simulink model "realistic_model"  (R2021b)
settings: Solver=VariableStepAuto  StartTime=0.0  StopTime=10  RelTol=1e-3
values from neighbouring files (symbols this model uses):
  A = [0 0 1 0 ... (first row only)    [main.m]
  B = [0 ... (first row only)    [main.m]
  C = [1 0 0 0 ... (first row only)    [main.m]
  K = K_temp    [main.m]    (also in plots_assignment2.m; plots_assignment3.m)
  Ts = 0.05    [main.m]
  Wc = wc_temp    (= 12.5663706144)    [main.m]    (also in plots_assignment3.m = wc_temp; tuning.m = 40.8407044967)
  x_initial = [0 0 0 0]'    [main.m]    (also in tuning.m)
settings Model: Creator=Marius  LastModifiedBy=Marius

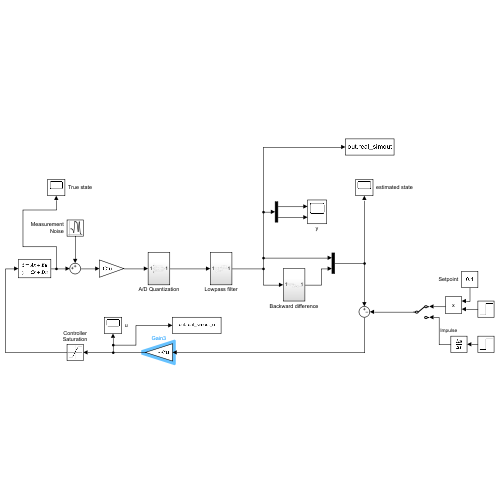
[thumbnail: Simulink's stored preview of the top-level diagram]
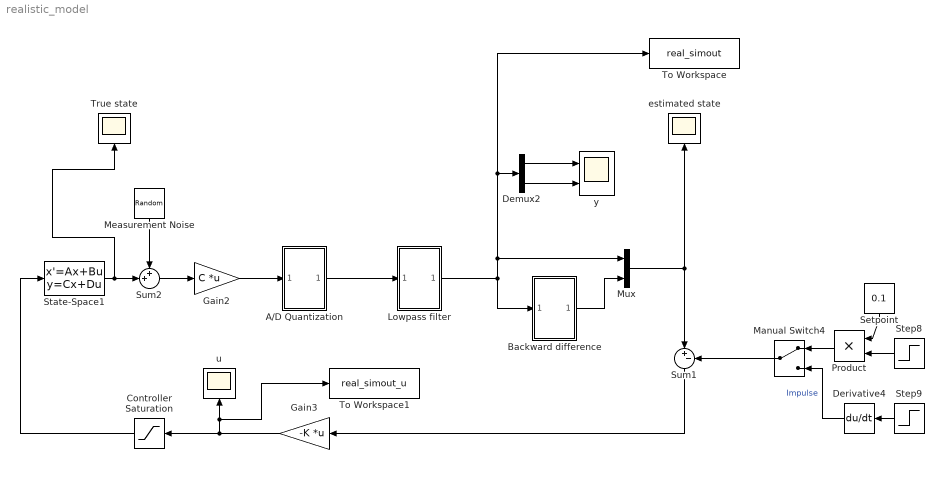
== system realistic_model ==
  A/D Quantization : Subsystem
  Backward difference : Subsystem
  Controller Saturation : Saturate  UpperLimit=5  LowerLimit=-5
  Demux2 : Demux  Outputs=2
  Derivative4 : Derivative
  Gain2 : Gain  Gain=C  Multiplication=Matrix(K*u)
  Gain3 : Gain  Gain=-K  Multiplication=Matrix(K*u)
  Lowpass filter : Subsystem
  Manual Switch4 : ManualSwitch
  Measurement Noise : RandomNumber  Mean=[0 0 0 0]  Variance=[0.0005 pi/1800 0 0].^2  SampleTime=0.1
  Mux : Mux  Inputs=2
  Product : Product
  Setpoint : Constant  Value=0.1
  State-Space1 : StateSpace  A=A  B=B  C=eye(4)  D=zeros(4,1)  InitialCondition=x_initial
  Step8 : Step  Before=[0 0 0 0]  After=[1 0 0 0]  SampleTime=0
  Step9 : Step  Before=[0 0 0 0]  After=[10 0 0 0]  SampleTime=0
  Sum1 : Sum  Inputs=|+-
  Sum2 : Sum  Inputs=++|
  To Workspace : ToWorkspace  VariableName=real_simout  SaveFormat=Timeseries  SampleTime=-1
  To Workspace1 : ToWorkspace  VariableName=real_simout_u  SaveFormat=Timeseries  SampleTime=-1
  True state : Scope
  estimated state : Scope
  u : Scope
  y : Scope  NumInputPorts=2
  wires:
  Manual Switch4/1 -> Sum1/2
  Gain3/1 -> Controller Saturation/1, To Workspace1/1, u/1
  Sum1/1 -> Gain3/1
  Demux2/2 -> y/2
  Demux2/1 -> y/1
  Step9/1 -> Derivative4/1
  Derivative4/1 -> Manual Switch4/2  "Impulse"
  Mux/1 -> estimated state/1, Sum1/1
  State-Space1/1 -> True state/1, Sum2/2
  Sum2/1 -> Gain2/1
  Measurement Noise/1 -> Sum2/1
  Backward difference/1(Out1) -> Mux/2
  Lowpass filter/1(Out1) -> Backward difference/1(In1), To Workspace/1, Demux2/1, Mux/1
  A/D Quantization/1(Out1) -> Lowpass filter/1(In1)
  Gain2/1 -> A/D Quantization/1(In1)
  Product/1 -> Manual Switch4/1
  Step8/1 -> Product/2
  Setpoint/1 -> Product/1
  Controller Saturation/1 -> State-Space1/1

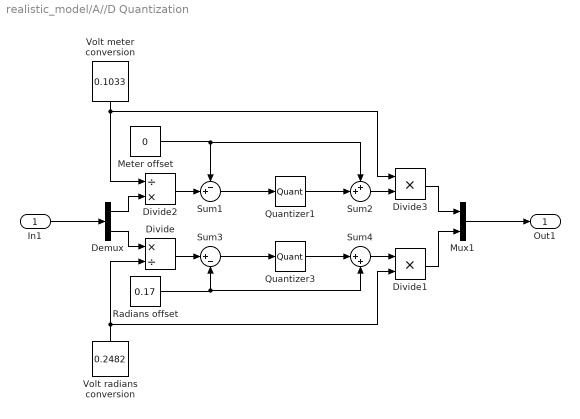
== system realistic_model/A//D Quantization ==
  In1 : Inport
  Demux : Demux  Outputs=2
  Divide : Product  Inputs=*/
  Divide1 : Product  Inputs=**
  Divide2 : Product  Inputs=/*
  Divide3 : Product  Inputs=**
  Meter offset : Constant  Value=0
  Mux1 : Mux  Inputs=2
  Quantizer1 : Quantizer  QuantizationInterval=20/2^16
  Quantizer3 : Quantizer  QuantizationInterval=20/2^16
  Radians offset : Constant  Value=0.17
  Sum1 : Sum  Inputs=-+|
  Sum2 : Sum  Inputs=++|
  Sum3 : Sum  Inputs=|+-
  Sum4 : Sum  Inputs=|++
  Volt meter conversion : Constant  Value=0.1033
  Volt radians conversion : Constant  Value=0.2482
  Out1 : Outport
  wires:
  Radians offset/1 -> Sum4/2, Sum3/2
  Quantizer3/1 -> Sum4/1
  Sum3/1 -> Quantizer3/1
  In1/1 -> Demux/1
  Mux1/1 -> Out1/1
  Divide/1 -> Sum3/1
  Demux/2 -> Divide/1
  Volt radians conversion/1 -> Divide1/2, Divide/2
  Sum4/1 -> Divide1/1
  Divide1/1 -> Mux1/2
  Divide3/1 -> Mux1/1
  Sum1/1 -> Quantizer1/1
  Quantizer1/1 -> Sum2/2
  Sum2/1 -> Divide3/2
  Divide2/1 -> Sum1/2
  Demux/1 -> Divide2/2
  Meter offset/1 -> Sum2/1, Sum1/1
  Volt meter conversion/1 -> Divide3/1, Divide2/1

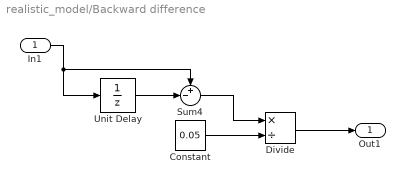
== system realistic_model/Backward difference ==
  In1 : Inport
  Constant : Constant  Value=0.05
  Divide : Product  Inputs=*/
  Sum4 : Sum  Inputs=+-|
  Unit Delay : UnitDelay  SampleTime=0.05  HasFrameUpgradeWarning=on
  Out1 : Outport
  wires:
  Divide/1 -> Out1/1
  In1/1 -> Sum4/1, Unit Delay/1
  Unit Delay/1 -> Sum4/2
  Constant/1 -> Divide/2
  Sum4/1 -> Divide/1

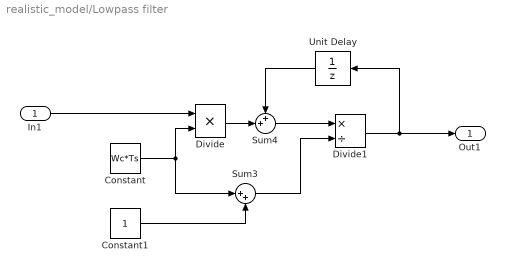
== system realistic_model/Lowpass filter ==
  In1 : Inport
  Constant : Constant  Value=Wc*Ts
  Constant1 : Constant
  Divide : Product  Inputs=**
  Divide1 : Product  Inputs=*/
  Sum3 : Sum  Inputs=|++
  Sum4 : Sum  Inputs=++|
  Unit Delay : UnitDelay  SampleTime=Ts  HasFrameUpgradeWarning=on
  Out1 : Outport
  wires:
  Divide/1 -> Sum4/2
  Divide1/1 -> Out1/1, Unit Delay/1
  Sum4/1 -> Divide1/1
  Sum3/1 -> Divide1/2
  Constant/1 -> Sum3/1, Divide/2
  Constant1/1 -> Sum3/2
  In1/1 -> Divide/1
  Unit Delay/1 -> Sum4/1
